simulink model "model"  (R2021b)
settings: Solver=VariableStepAuto  StartTime=0.0  StopTime=10.0  RelTol=1e-3
undefined symbols (not defined in the file): Newton, Raphson
settings Model: Creator=O  LastModifiedBy=wangzixuan

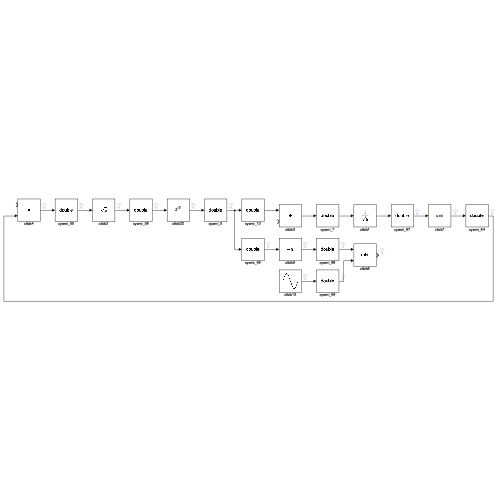
[thumbnail: Simulink's stored preview of the top-level diagram]
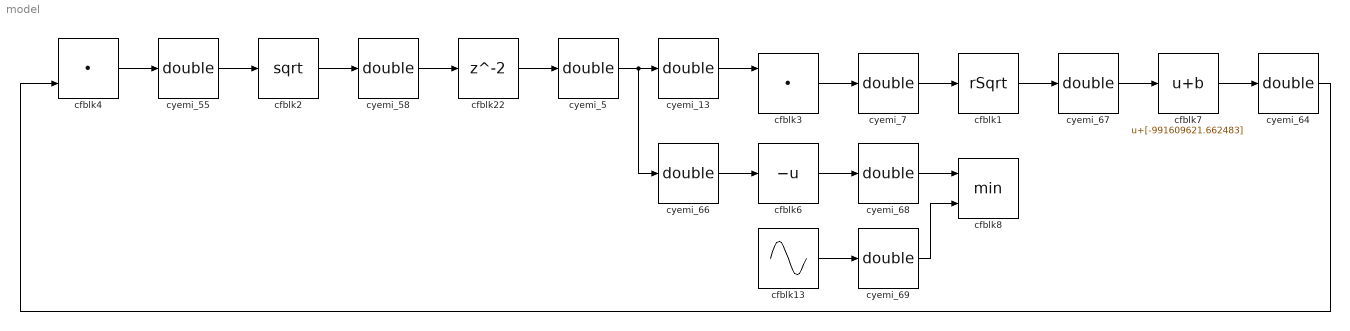
== system model ==
  cfblk1 : Sqrt  Operator=rSqrt  OutDataTypeStr=double  AlgorithmType=Newton-Raphson  SaturateOnIntegerOverflow=on
  cfblk13 : Sin  Amplitude=[-506831533.045897]  Bias=[-374132303.029973]  SampleTime=0
  cfblk2 : Sqrt  OutDataTypeStr=double  SaturateOnIntegerOverflow=on
  cfblk22 : Delay  SampleTime=1
  cfblk3 : DotProduct  OutDataTypeStr=double  InputSameDT=on
  cfblk4 : DotProduct  OutDataTypeStr=double  InputSameDT=on
  cfblk6 : UnaryMinus
  cfblk7 : Bias  Bias=[-991609621.662483]
  cfblk8 : MinMax  Inputs=2  OutDataTypeStr=double
  cyemi_{5,7,13,55,58,64,66..69} (10 alike) : DataTypeConversion  OutDataTypeStr=double
  wires:
  cfblk7/1 -> cyemi_64/1
  cfblk4/1 -> cyemi_55/1
  cfblk13/1 -> cyemi_69/1
  cyemi_69/1 -> cfblk8/2
  cfblk2/1 -> cyemi_58/1
  cyemi_67/1 -> cfblk7/1
  cyemi_64/1 -> cfblk4/2
  cfblk1/1 -> cyemi_67/1
  cfblk6/1 -> cyemi_68/1
  cyemi_5/1 -> cyemi_13/1, cyemi_66/1
  cyemi_55/1 -> cfblk2/1
  cyemi_66/1 -> cfblk6/1
  cyemi_58/1 -> cfblk22/1
  cfblk3/1 -> cyemi_7/1
  cfblk22/1 -> cyemi_5/1
  cyemi_7/1 -> cfblk1/1
  cyemi_68/1 -> cfblk8/1
  cyemi_13/1 -> cfblk3/1
